simulink model "estimate1"  (Simulink 4.00)
settings: Solver=ode45  StartTime=0.0  StopTime=20.0  RelTol=1e-3
values from neighbouring files (symbols this model uses):
  a = [-0.5, 0, 0; 0, -3, 0; 0, 0, -6]    [estimate_1.m]    (also in estimate_2.m; estimate_3.m; estimate_31.m; pol1.m = real(s1))
  b = [0, 0; 1, 0; 0, 1]    [estimate_1.m]    (also in estimate_2.m; estimate_3.m; estimate_31.m; pol1.m = imag(s1))
  c = [0.3, 0.5, 1]    [estimate_1.m]    (also in estimate_2.m; estimate_3.m; estimate_31.m)
  dt = 0.1    [estimate_1.m]    (also in estimate_2.m; estimate_3.m; estimate_31.m; kalm1.m)
  x0 = [5, 0, 0, 0]    [abeob1.m]    (also in alqr1.m; alqrd1.m; apol1.m; estimate_1.m = [1 2 3])
libraries: simulink3 x1, cstblocks x1
settings Model: LastModifiedBy=Administrator  BlockReductionOpt=off

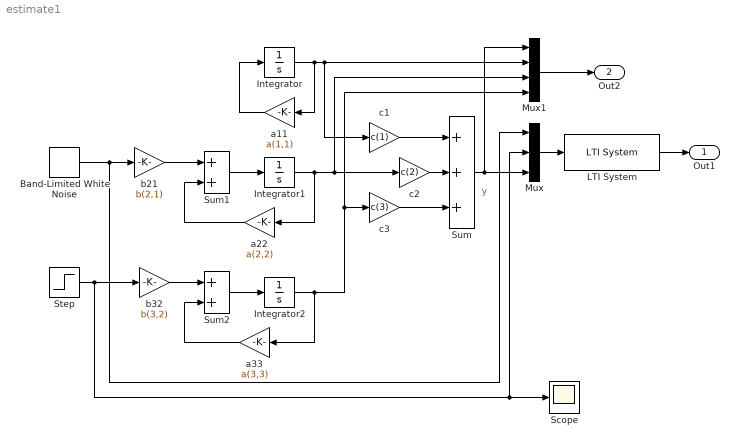
== system estimate1 ==
  note: y
  Band-Limited White Noise : simulink3/Sources/Band-Limited White Noise  Cov=[dt]  Ts=dt  seed=[23341]
  Integrator : Integrator  ExternalReset=none  InitialConditionSource=internal  InitialCondition=x0(1)  LimitOutput=off  UpperSaturationLimit=inf  LowerSaturationLimit=-inf  ShowSaturationPort=off  ShowStatePort=off  AbsoluteTolerance=auto
  Integrator1 : Integrator  ExternalReset=none  InitialConditionSource=internal  InitialCondition=x0(2)  LimitOutput=off  UpperSaturationLimit=inf  LowerSaturationLimit=-inf  ShowSaturationPort=off  ShowStatePort=off  AbsoluteTolerance=auto
  Integrator2 : Integrator  ExternalReset=none  InitialConditionSource=internal  InitialCondition=x0(3)  LimitOutput=off  UpperSaturationLimit=inf  LowerSaturationLimit=-inf  ShowSaturationPort=off  ShowStatePort=off  AbsoluteTolerance=auto
  LTI System : cstblocks/LTI System  sys=my_estim  IC=0
  Mux : Mux  Inputs=3
  Mux1 : Mux  Inputs=4
  Scope : Scope
      settings: TimeRange=auto  YMin=-5  YMax=5  SaveToWorkspace=off  SaveName=ScopeData  LimitDataPoints=on  MaxDataPoints=5000
  Step : Step  Time=0  Before=0  After=1  SampleTime=0
  Sum : Sum  Inputs=+++  SaturateOnIntegerOverflow=on
  Sum1 : Sum  Inputs=++  SaturateOnIntegerOverflow=on
  Sum2 : Sum  Inputs=++  SaturateOnIntegerOverflow=on
  a11 : Gain  Orientation=left  Gain=a(1,1)  Multiplication=Element-wise(K.*u)  SaturateOnIntegerOverflow=on
  a22 : Gain  Orientation=left  Gain=a(2,2)  Multiplication=Element-wise(K.*u)  SaturateOnIntegerOverflow=on
  a33 : Gain  Orientation=left  Gain=a(3,3)  Multiplication=Element-wise(K.*u)  SaturateOnIntegerOverflow=on
  b21 : Gain  Gain=b(2,1)  Multiplication=Element-wise(K.*u)  SaturateOnIntegerOverflow=on
  b32 : Gain  Gain=b(3,2)  Multiplication=Element-wise(K.*u)  SaturateOnIntegerOverflow=on
  c1 : Gain  Gain=c(1)  Multiplication=Element-wise(K.*u)  SaturateOnIntegerOverflow=on
  c2 : Gain  Gain=c(2)  Multiplication=Element-wise(K.*u)  SaturateOnIntegerOverflow=on
  c3 : Gain  Gain=c(3)  Multiplication=Element-wise(K.*u)  SaturateOnIntegerOverflow=on
  Out1 : Outport  Port=1
  Out2 : Outport  Port=2
  wires:
  a11/1 -> Integrator/1
  Integrator/1 -> a11/1, Mux1/2, c1/1
  Integrator1/1 -> a22/1, Mux1/3, c2/1
  Sum1/1 -> Integrator1/1
  a22/1 -> Sum1/2
  Band-Limited White Noise/1 -> b21/1, Mux/1
  b21/1 -> Sum1/1
  Integrator2/1 -> a33/1, Mux1/4, c3/1
  Sum2/1 -> Integrator2/1
  a33/1 -> Sum2/2
  Step/1 -> b32/1, Mux/2, Scope/1
  b32/1 -> Sum2/1
  Mux/1 -> LTI System/1
  LTI System/1 -> Out1/1
  Mux1/1 -> Out2/1
  Sum/1 -> Mux/3, Mux1/1
  c1/1 -> Sum/1
  c2/1 -> Sum/2
  c3/1 -> Sum/3
